simulink model "Copy_of_cart_pole_SMC"  (R2020b)
settings: Solver=VariableStepAuto  StartTime=0.0  StopTime=10.0  RelTol=1e-3
settings Model: Creator=Taha  LastModifiedBy=Taha

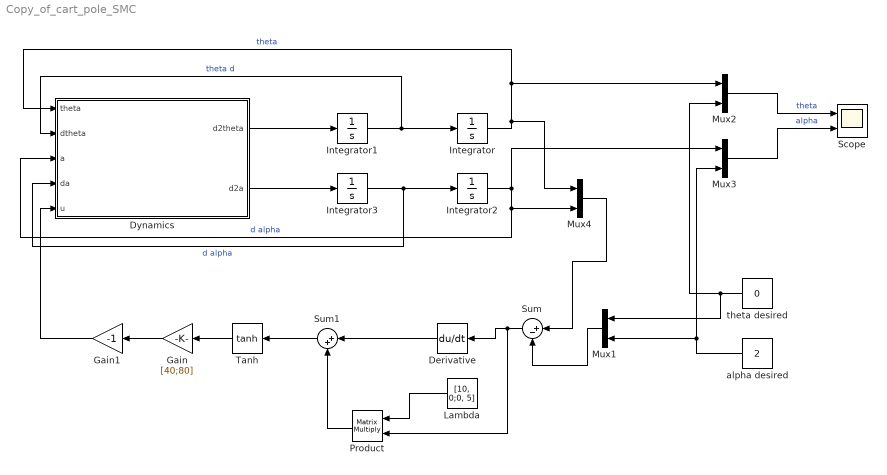
== system Copy_of_cart_pole_SMC ==
  Derivative : Derivative
  Dynamics : MATLAB Function  TreatAsAtomicUnit=on
  Gain : Gain  Gain=[40;80]
  Gain1 : Gain  Gain=-1
  Integrator : Integrator  InitialCondition=randn  ContinuousStateAttributes='theta'
  Integrator1 : Integrator
  Integrator2 : Integrator  InitialCondition=randn  ContinuousStateAttributes='alpha'
  Integrator3 : Integrator
  Lambda : Constant  Value=[10, 0;0, 5]
  Mux{1..4} (4 alike) : Mux  Inputs=2
  Product : Product  Multiplication=Matrix(*)
  Scope : Scope  NumInputPorts=2
  Sum : Sum  Inputs=|+-
  Sum1 : Sum  Inputs=|++
  Tanh : Trigonometry  Operator=tanh
  alpha desired : Constant  Value=2
  theta desired : Constant  Value=0
  wires:
  Integrator1/1 -> Dynamics/2(dtheta), Integrator/1  "theta d"
  Dynamics/2(d2a) -> Integrator3/1
  Dynamics/1(d2theta) -> Integrator1/1
  Integrator3/1 -> Dynamics/4(da), Integrator2/1  "d alpha"
  Integrator2/1 -> Mux4/2, Dynamics/3(a), Mux3/1  "d alpha"
  Integrator/1 -> Mux4/1, Dynamics/1(theta), Mux2/1  "theta"
  theta desired/1 -> Mux1/1, Mux2/2
  alpha desired/1 -> Mux1/2, Mux3/2
  Derivative/1 -> Sum1/1
  Lambda/1 -> Product/1
  Product/1 -> Sum1/2
  Sum1/1 -> Tanh/1
  Tanh/1 -> Gain/1
  Gain/1 -> Gain1/1
  Gain1/1 -> Dynamics/5(u)
  Mux2/1 -> Scope/1  "theta"
  Mux3/1 -> Scope/2  "alpha"
  Mux4/1 -> Sum/1
  Mux1/1 -> Sum/2
  Sum/1 -> Product/2, Derivative/1

== matlab function Copy_of_cart_pole_SMC/Dynamics ==
  data: theta input; dtheta input; d2theta output; d2a output; a input; da input; u input
function [d2theta,d2a ] = fcn(theta, dtheta, a, da, u)

A = 3.291;
B = 0.12519;
C = 0.23688;
D = 6.0521;

% A = 0.1266
% B = 0.0118;
% C = 0.4683;
% D = 422.5586;


d2theta = (-A * B * sin(a) * cos(a)^2 * dtheta^2 ...
    + A * C * sin(a) * cos(a) ...
    -2 * B^2 * sin(a) * cos(a) * da * dtheta ...
    + A * B * sin(a) * da^2 ...
    + B * u) ...
    / (B^2 * sin(a)^2 * a + B * D - A^2 * cos(a)^2 * a);



d2a = ( 2 * A * B * sin(a) * cos(a)^2 * dtheta * da ...
    -A^2 * sin(a) * cos(a) * da^2 ...
    + B^2 * sin(a)^3 * cos(a) * dtheta^2 ...
    + theta * C * sin(a) * cos(a) * dtheta^2 ...
    - B * C * sin(a)^3 ...
    - D * C * sin(a) ...
    - A * cos(a) * u)...
    / (B^2 * sin(a)^2 ...
    + B * C ...
    - A^2 * cos(a)^2);
